simulink model "pendule_inv_etu"  (R2022b)
settings: Solver=VariableStepAuto  StartTime=0.0  StopTime=10.0  RelTol=1e-3
values from neighbouring files (symbols this model uses):
  g = 9.81    [simu_pendule_inv_capteur_etu.m]    (also in simu_pendule_inv_etu.m)
  K = [10 1]    [simu_pendule_inv_capteur_etu.m]    (also in simu_pendule_inv_etu.m = [30 10])
  l = 10    [simu_pendule_inv_capteur_etu.m]    (also in simu_pendule_inv_etu.m)
  ue = 0    [simu_pendule_inv_capteur_etu.m]    (also in simu_pendule_inv_etu.m)
  x0 = [pi/20 0]'    [simu_pendule_inv_capteur_etu.m]    (also in simu_pendule_inv_etu.m = [pi/10 0]')
  xe = [0 0]'    [simu_pendule_inv_capteur_etu.m]    (also in simu_pendule_inv_etu.m)
settings Model: Creator=marga  LastModifiedBy=marga

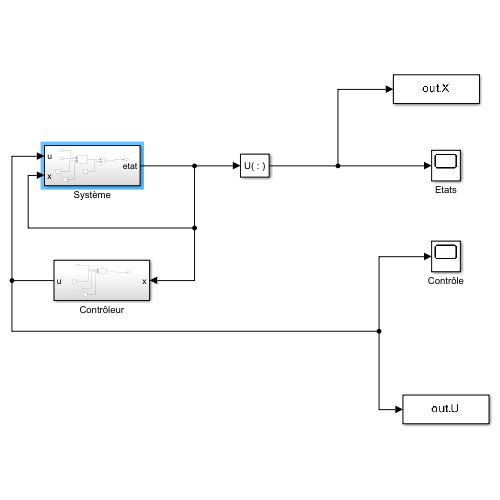
[thumbnail: Simulink's stored preview of the top-level diagram]
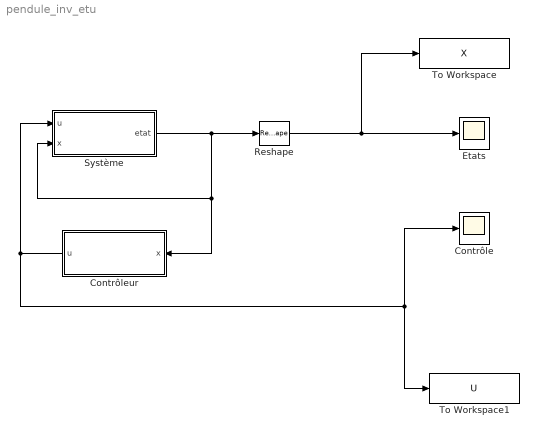
== system pendule_inv_etu ==
  Contrôle : Scope
  Contrôleur : Subsystem
  Etats : Scope
  Reshape : Reshape
  Système : Subsystem
  To Workspace : ToWorkspace  VariableName=X  SaveFormat=Timeseries  SampleTime=-1
  To Workspace1 : ToWorkspace  VariableName=U  SaveFormat=Timeseries  SampleTime=-1
  wires:
  Système/1(etat) -> Système/2(x), Contrôleur/1(x), Reshape/1
  Contrôleur/1(u) -> Contrôle/1, To Workspace1/1, Système/1(u)
  Reshape/1 -> To Workspace/1, Etats/1

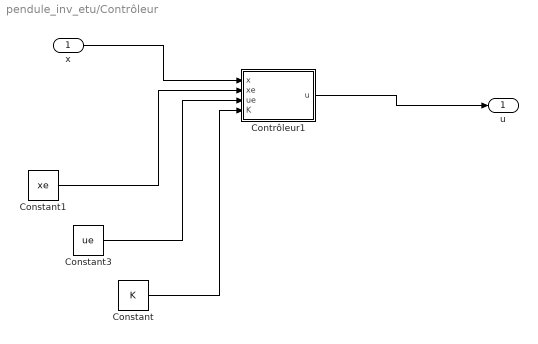
== system pendule_inv_etu/Contrôleur ==
  x : Inport
  Constant : Constant  Value=K  VectorParams1D=off
  Constant1 : Constant  Value=xe
  Constant3 : Constant  Value=ue
  Contrôleur1 : MATLAB Function  TreatAsAtomicUnit=on
  u : Outport
  wires:
  Constant1/1 -> Contrôleur1/2(xe)
  Constant3/1 -> Contrôleur1/3(ue)
  x/1 -> Contrôleur1/1(x)
  Constant/1 -> Contrôleur1/4(K)
  Contrôleur1/1(u) -> u/1

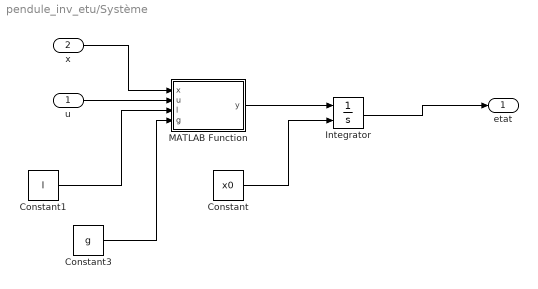
== system pendule_inv_etu/Système ==
  u : Inport
  x : Inport  Port=2
  Constant : Constant  Value=x0
  Constant1 : Constant  Value=l
  Constant3 : Constant  Value=g
  Integrator : Integrator  InitialConditionSource=external
  MATLAB Function : MATLAB Function  TreatAsAtomicUnit=on
  etat : Outport
  wires:
  MATLAB Function/1(y) -> Integrator/1
  Integrator/1 -> etat/1
  u/1 -> MATLAB Function/2(u)
  Constant/1 -> Integrator/2
  Constant1/1 -> MATLAB Function/3(l)
  Constant3/1 -> MATLAB Function/4(g)
  x/1 -> MATLAB Function/1(x)

== matlab function pendule_inv_etu/Système/MATLAB Function ==
  data: x input; u input; y output; l input; g input
function y = fcn(x,u,l,g)

y = [x(2) g/l*sin(x(1))-u/l*cos(x(1))];

== matlab function pendule_inv_etu/Contrôleur/Contrôleur1 ==
  data: x input; u output; xe input; ue input; K input
function u = fcn(x,xe,ue,K)

u = ue + K*(x-xe);
